simulink model "RefModel_VisualLanding"  (R2020b)
settings: Solver=ode1  StartTime=0.0  StopTime=inf  FixedStep=Ts_VisualLanding.Ts_Base  RelTol=1e-3
values from neighbouring files (symbols this model uses):
  VISLANDING_PARAM_V10 = VISLANDING_PARAM_V1000    [INIT_VisualLanding.m]    (also in SetAlgoParam_VisualLanding.m)
  VISLANDING_PARAM_V1000 = Simulink.Bus.createMATLABStruct('BUS_VISUALLANDING_PARAM')    [INIT_VisualLanding.m]    (also in SetAlgoParam_VisualLanding.m)
settings Model: PauseTimes=[308,310,12]  Creator=sl  LastModifiedBy=sl
settings DataIOCC: SaveOutput=off  SaveTime=off
settings OptimizationCC: DefaultParameterBehavior=Inlined  EnhancedBackFolding=on  PassReuseOutputArgsAs=Individual arguments  ZeroExternalMemoryAtStartup=off  ZeroInternalMemoryAtStartup=off  OptimizeBlockOrder=speed  DifferentSizesBufferReuse=on  OptimizationCustomize=off  EfficientTunableParamExpr=on
settings DebuggingCC: InheritedTsInSrcMsg=none  ParameterPrecisionLossMsg=none  ParameterTunabilityLossMsg=error  UnconnectedInputMsg=none  UnconnectedOutputMsg=none  UnconnectedLineMsg=none  SFUnusedDataAndEventsDiag=none
settings HardwareCC: ProdBitPerPointer=32  ProdBitPerSizeT=32  ProdBitPerPtrDiffT=32  ProdLargestAtomicInteger=Long  ProdLargestAtomicFloat=Double  ProdWordSize=32  ProdHWDeviceType=ARM Compatible->ARM Cortex
settings ModelReferenceCC: ModelReferenceNumInstancesAllowed=Single
settings SFSimCC: MATLABDynamicMemAlloc=off
settings RTWCC: Description=Embedded Coder  SystemTargetFile=ert.tlc  TemplateMakefile=ert_default_tmf  GenerateReport=on  IncludeHyperlinkInReport=on  LaunchReport=on  GenerateTraceInfo=on  GenerateTraceReport=on  GenerateTraceReportSl=on  GenerateTraceReportSf=on  GenerateTraceReportEml=on
settings CodeAppCC: ForceParamTrailComments=on  IgnoreCustomStorageClasses=off  MaxIdLength=48  OperatorAnnotations=on  SimulinkDataObjDesc=on  SFDataObjDesc=on  InsertBlockDesc=on
settings ERTTargetCC: TargetLangStandard=C99 (ISO)  GenerateSampleERTMain=on  CombineOutputUpdateFcns=off  LogVarNameModifier=none  SupportVariableSizeSignals=on  InlinedParameterPlacement=NonHierarchical  ERTCustomFileTemplate=example_file_process.tlc

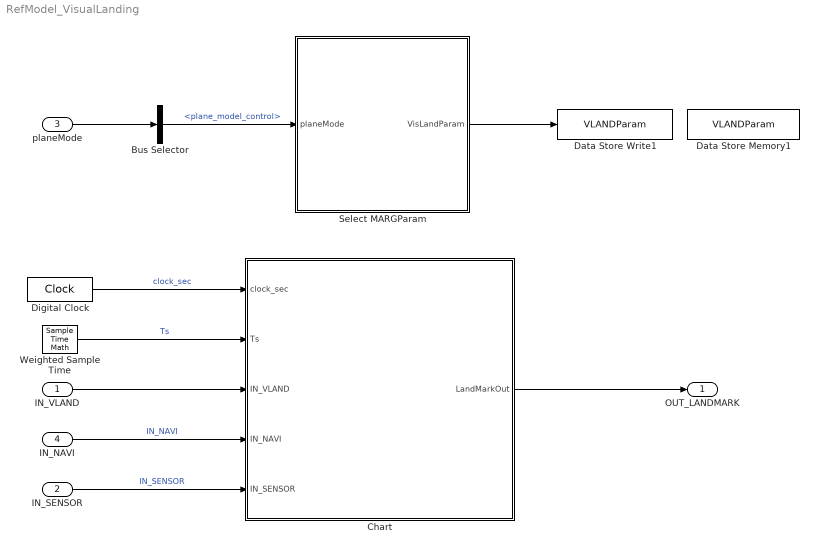
== system RefModel_VisualLanding ==
  IN_VLAND : Inport  OutDataTypeStr=Bus: BUS_VISUALLANDING_INPUT  PortDimensions=1  BusOutputAsStruct=on
  IN_SENSOR : Inport  Port=2  OutDataTypeStr=Bus: BUS_SENSOR  BusOutputAsStruct=on
  planeMode : Inport  Port=3  OutDataTypeStr=Bus: BUS_SYSTEMINFO_INPUT
  IN_NAVI : Inport  Port=4  OutDataTypeStr=Bus: BUS_NAVI_TO_FIRM  BusOutputAsStruct=on
  Bus Selector : BusSelector  OutputSignals=plane_model_control
  Chart : Stateflow chart  TreatAsAtomicUnit=on
  Data Store Memory1 : DataStoreMemory  DataStoreName=VLANDParam  ReadBeforeWriteMsg=warning  WriteAfterWriteMsg=warning  WriteAfterReadMsg=warning  ShowAdditionalParam=off  OutDataTypeStr=Bus: BUS_VISUALLANDING_PARAM  Dimensions=1
  Data Store Write1 : DataStoreWrite  DataStoreName=VLANDParam
  Digital Clock : DigitalClock  SampleTime=-1
  Select MARGParam : Subsystem
  Weighted Sample Time : SampleTimeMath  TsampMathOp=Ts Only
  OUT_LANDMARK : Outport  OutDataTypeStr=Bus: BUS_VISUALLANDING_LANDMARK
  wires:
  IN_VLAND/1 -> Chart/3(IN_VLAND)
  IN_NAVI/1 -> Chart/4(IN_NAVI)  "IN_NAVI"
  IN_SENSOR/1 -> Chart/5(IN_SENSOR)  "IN_SENSOR"
  Bus Selector/1 -> Select MARGParam/1(planeMode)  "<plane_model_control>"
  Select MARGParam/1(VisLandParam) -> Data Store Write1/1
  planeMode/1 -> Bus Selector/1
  Chart/1(LandMarkOut) -> OUT_LANDMARK/1
  Weighted Sample Time/1 -> Chart/2(Ts)  "Ts"
  Digital Clock/1 -> Chart/1(clock_sec)  "clock_sec"

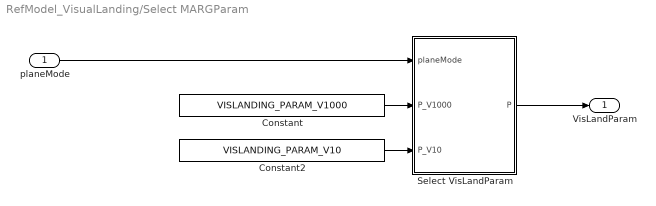
== system RefModel_VisualLanding/Select MARGParam ==
  planeMode : Inport
  Constant : Constant  Value=VISLANDING_PARAM_V1000  OutDataTypeStr=Bus: BUS_VISUALLANDING_PARAM
  Constant2 : Constant  Value=VISLANDING_PARAM_V10  OutDataTypeStr=Bus: BUS_VISUALLANDING_PARAM
  Select VisLandParam : MATLAB Function  TreatAsAtomicUnit=on
  VisLandParam : Outport
  wires:
  Constant/1 -> Select VisLandParam/2(P_V1000)
  Constant2/1 -> Select VisLandParam/3(P_V10)
  Select VisLandParam/1(P) -> VisLandParam/1
  planeMode/1 -> Select VisLandParam/1(planeMode)

== matlab function RefModel_VisualLanding/Select MARGParam/Select VisLandParam ==
  data: planeMode input Enum: ENUM_plane_mode; P output Bus: BUS_VISUALLANDING_PARAM; P_V1000 input Bus: BUS_VISUALLANDING_PARAM; P_V10 input Bus: BUS_VISUALLANDING_PARAM
function P = fcn(planeMode,P_V1000,P_V10)
switch planeMode
    case ENUM_plane_mode.V10
        P = P_V10;
    case {ENUM_plane_mode.V1000,ENUM_plane_mode.V10s}
        P = P_V1000;
    otherwise
        P = P_V1000;
end

== stateflow chart RefModel_VisualLanding/Chart ==
  state Calculate [parallel]
    en:
    initLandMarkOut();
    du:
    algebraMethod();
    if VLANDParam.enableStateEstimate
    LandMarkOut.estMode = ENUM_EstModeVisLand.StateEstimate;
    KalmanFilterMethod();
    end
    predictLLA();
    settings: executionOrder=2
  state Status [parallel]
    settings: executionOrder=1
    state updateFlag [parallel]
      en:
      du:
      updateRefreshFlag();
      settings: executionOrder=1
    state ValidFlag [parallel]
      en:
      du:
      updateVLFlag();
      settings: executionOrder=2
  data: x_out function_output; pos_landmark function_input; vel_uav function_input; pos_uav function_input; Ts_in function_input; P_out function_output; dz_out function_output; Pz_out function_output; reset function_input; reject_threshold function_input; Q function_input; R function_input; mode function_input; clock_sec input; Ts input; IN_VLAND input; IN_NAVI input; IN_SENSOR input; VLANDParam data_store_memory; LandMarkOut output Bus: BUS_VISUALLANDING_LANDMARK size=1
  function updateRefreshFlag:
    | function updateRefreshFlag
    | % 判断数据更新时刻
    | persistent lastValidIdx preIdx
    | idxAll = IN_VLAND.idxAll;
    | if isempty(lastValidIdx)
    |     lastValidIdx = idxAll;
    |     preIdx = idxAll;
    | end
    | curIdx = idxAll;
    | if preIdx ~= curIdx
    |     LandMarkOut.updateFlag = true;
    | else
    |     LandMarkOut.updateFlag = false;
    | end
    | preIdx = idxAll;
  function algebraMethod:
    | function algebraMethod
    | % c: 相机坐标系 camera
    | % l: 着陆标志坐标系 landmark
    | % b: 机体坐标系 body
    | % e: NED坐标系 
    | % cl: landing mark to camera
    | % be: ned to body
    | % cb: body to camera
    | %%
    | if IN_VLAND.nDetect ~= 0 && LandMarkOut.updateFlag% 检测到至少1个tag
    |     tcl = getTcl(IN_VLAND);
    |     [Rcl,eulerd] = getRcl(IN_VLAND); 
    |     Rcb = VLANDParam.Rcb;
    |     Rbc = Rcb';
    |     Rbe = calRbe(double(IN_NAVI.eulerd_yaw_pitch_roll)*pi/180);
    |     Rlc = Rcl';
    |     Rce = Rcb*Rbe;
    |     Rec = Rce';
    |     Rle = Rlc*Rcb*Rbe;
    |     Rel = Rle';
    | 
    |     pos_uav = double(IN_NAVI.posNED);
    |     lla_uav = IN_NAVI.lla;
    | 
    |     LandMarkOut.Rcl = Rcl;
    |     LandMarkOut.Rbl = Rbe*Rel;
    |     LandMarkOut.Rel = Rel;
    | 
    |     LandMarkOut.Pc = tcl; % 路标中心相对相机中心的位置矢量，在相机坐标系中表示
    |     
    |     LandMarkOut.Pe = Rec * LandMarkOut.Pc + pos_uav;
    |     LandMarkOut.Pb = Rbc * LandMarkOut.Pc;
    | 
    |     LandMarkOut.estMode = ENUM_EstModeVisLand.Geometry;
    |     
    |     relPosNED = Rec * LandMarkOut.Pc;
    |     dlat = 1/111e3*relPosNED(1);
    |     dlon = 1/cos(IN_NAVI.lla(1)*pi/180)/111e3*relPosNED(2);
    |     dh = -relPosNED(3);
    |     LandMarkOut.LLA = lla_uav + [dlat;dlon;dh];
    | end
    | end
    | % LandMarkOut.Ve = [0;0;0];
    | %%
    | % 计算Rbe
    | function out = calRbe(euler_yaw_pitch_roll)
    | yaw_be = euler_yaw_pitch_roll(1);
    | pitch_be = euler_yaw_pitch_roll(2);
    | roll_be = euler_yaw_pitch_roll(3);
    | out = Rzyx(yaw_be,pitch_be,roll_be);
    | end
    | % 计算平均tcl
    | function tcl = getTcl(IN_VLAND)
    | if IN_VLAND.Tagl.isDetect
    |     tcl = IN_VLAND.Tagl.tcl;
    | elseif IN_VLAND.Tagm.isDetect
    |     tcl = IN_VLAND.Tagm.tcl; 
    | else
    |     tcl = IN_VLAND.Tags.tcl;
    | end
    | end
    | % 计算平均Rcl
    | function [Rcl,eulerd] = getRcl(IN_VLAND)
    | if IN_VLAND.Tagl.isDetect
    |     Rcl = IN_VLAND.Tagl.Rcl;
    |     eulerd = IN_VLAND.Tagl.eulerdcl;
    | elseif IN_VLAND.Tagm.isDetect
    |     Rcl = IN_VLAND.Tagm.Rcl; 
    |     eulerd = IN_VLAND.Tagl.eulerdcl;
    | else
    |     Rcl = IN_VLAND.Tags.Rcl;
    |     eulerd = IN_VLAND.Tagl.eulerdcl;
    | end
    | % Rcl = double(Rcl);
    | % eulerd = double(eulerd);
    | end
  function [x_out,P_out,dz_out,Pz_out] = landmarkKF(pos_landmark, vel_uav, pos_uav, Ts_in,reset,reject_threshold,Q,R,mode):
    | function [x_out,P_out,dz_out,Pz_out] = landmarkKF(pos_landmark, vel_uav, pos_uav, Ts_in,reset,reject_threshold,Q,R,mode)
    | persistent x P dz Pz
    | pos_landmark0 = reshape(pos_landmark,[3,1]);
    | if isempty(x) || reset
    |     vel_landmark0 = [0;0;0];
    |     state0 = [pos_landmark0;vel_landmark0];
    |     x = state0;
    |     P = diag([3^2*ones(3,1);10^2*ones(3,1);]);
    |     
    |     dz = zeros(3,1);
    |     Pz = zeros(3,3);
    | end
    | 
    | switch mode
    |     case 'predict'
    |         % 预测
    |         u = [0;0;0];
    |         [x,P] = predict(x,u,Ts_in,P,Q);
    |     otherwise % 'fuse'
    |         % 矫正
    |         z = pos_landmark;
    |         [x,P,dz,Pz] = fusePos(x,z,P,R,reject_threshold);
    | end
    | x_out = x;
    | P_out = P;
    | dz_out = dz;
    | Pz_out = Pz;
    | %%
    | % 测量
    | function [z,H] = measure(x)
    | pos_lm = x(1:3);
    | z = pos_lm;
    | H = [1 0 0  0 0 0;
    |      0 1 0  0 0 0;
    |      0 0 1  0 0 0];
    | % 预测
    | function [x,P] = predict(x,u,Ts,P,Q)
    | pos_lm = x(1:3);
    | vel_lm = x(4:6);
    | pos_lm = pos_lm + vel_lm*Ts;
    | vel_lm = vel_lm + u;
    | x = [pos_lm;vel_lm];
    | A = [zeros(3,3)   eye(3,3);
    |      zeros(3,3) zeros(3,3);];
    | PHI = eye(6) + A*Ts;
    | P = PHI*P*PHI' + Q*Ts;
    | % 校正
    | function [x,P,dz,Pz] = fusePos(x,z,P,R,reject_threshold)
    | [z_prop,H] = measure(x);
    | dz = z - z_prop;
    | Pz = H*P*H'+R;
    | % if abs(dz) < reject_threshold
    |     % 残差小于阈值
    |     K = P*H'/(H*P*H'+R);
    |     P = (eye(size(K,1))-K*H)*P;
    |     P = (P+P')/2;
    |     x = x + K*dz;
    | % else
    | %     % 残差超限拒绝测量值
    | %     x = x;
    | %     P = P;
    | % end
  function updateVLFlag:
    | function updateVLFlag
    | % 更新视觉计算
    | persistent lastValidIdx preIdx sumInvalidIdx
    | idxAll = IN_VLAND.idxAll;
    | validFlag = IN_VLAND.validFlag;
    | frameRate = IN_VLAND.frameRate;
    | if isempty(lastValidIdx)
    |     lastValidIdx = idxAll;
    |     preIdx = idxAll;
    |     sumInvalidIdx = 0;
    | end
    | curIdx = idxAll;
    | if preIdx ~= curIdx
    |     updateFlag = true;
    | else
    |     updateFlag = false;
    | end
    | preIdx = idxAll;
    | if updateFlag % 当更新帧时进行一次检测有效性判定
    |     if ~validFlag
    |         sumInvalidIdx = sumInvalidIdx + 1;
    |     else
    |         sumInvalidIdx = 0;
    |     end
    | end
    | timeTh = 3*frameRate;
    | if sumInvalidIdx >= timeTh % 当连续出现N次检测不到tag时，认为跟踪失败
    |     LandMarkOut.validFlag = false;
    | else
    |     LandMarkOut.validFlag = true;
    | end
  function predictLLA:
    | function predictLLA
    | % 根据速度进行纬度、经度外推，高度不外推
    | if LandMarkOut.validFlag
    |     dposn_m = LandMarkOut.Ve(1)*Ts;
    |     dpose_m = LandMarkOut.Ve(2)*Ts;
    |     dlat = 1/111e3*dposn_m;
    |     dlon = 1/cos(IN_NAVI.lla(1)*pi/180)/111e3*dpose_m;
    |     dh = 0;
    |     LandMarkOut.LLA = LandMarkOut.LLA + [dlat;dlon;dh];
    | end
  function KalmanFilterMethod:
    | function KalmanFilterMethod
    | % persistent dz x P Pz
    | % if isempty(dz) ||...
    | %         ~LandMarkOut.validFlag % Tag跟踪丢失
    | %     dz = 0;
    | %     x = 0;
    | %     P = diag([]);
    | %     Pz = 0;
    | % end
    | persistent preValidFlag
    | if isempty(preValidFlag)
    |     preValidFlag = false;
    | end
    | if ~preValidFlag && LandMarkOut.validFlag
    |     resetKF = true;
    | else
    |     resetKF = false;
    | end
    | preValidFlag = LandMarkOut.validFlag;
    | %%
    | if LandMarkOut.validFlag
    |     pos_uav = double(IN_NAVI.posNED);
    |     vel_uav = double(IN_NAVI.velNED);
    |     pos_landmark = LandMarkOut.Pe;
    | 
    |     R = diag([1*ones(3,1)].^2); % 高度测量偏差
    |     sigma_pos_ml = 0.1*ones(3,1);
    |     sigma_vel_ml = 3*ones(3,1);
    |     Q = diag([sigma_pos_ml;sigma_vel_ml;].^2);
    |     reject_threshold = 0;
    |     % [x,P,dz,Pz] = landmarkKF(Vd,heightRadar1,Ts,resetKF,reject_threshold,Q,R,'predict');
    |     [x,P,dz,Pz] = landmarkKF(pos_landmark, vel_uav, pos_uav, Ts,resetKF,reject_threshold,Q,R,'predict');
    |     if LandMarkOut.updateFlag
    |         [x,P,dz,Pz] = landmarkKF(pos_landmark, vel_uav, pos_uav, Ts,resetKF,reject_threshold,Q,R,'fuse');
    |     end
    |     LandMarkOut.Pe = x(1:3);
    |     LandMarkOut.Ve = x(4:6);
    |     LandMarkOut.posCov = diag(P(1:3,1:3));
    |     LandMarkOut.velCov = diag(P(4:6,4:6));
    | else
    |     LandMarkOut.Ve = [0;0;0];
    | end
  function initLandMarkOut:
    | function initLandMarkOut
    | LandMarkOut.Rcl = zeros(3);
    | LandMarkOut.Rbl = zeros(3);
    | LandMarkOut.Rel = zeros(3);
    | 
    | LandMarkOut.LLA = zeros(3,1);
    | LandMarkOut.Pe = zeros(3,1);
    | LandMarkOut.Ve = zeros(3,1);
    | LandMarkOut.Pc = zeros(3,1); % 路标中心相对相机中心的位置矢量，在相机坐标系中表示
    | LandMarkOut.Pb = zeros(3,1);
    | LandMarkOut.posCov = zeros(3,1);
    | LandMarkOut.velCov = zeros(3,1);
    | LandMarkOut.estMode = ENUM_EstModeVisLand.Geometry;
    | LandMarkOut.validFlag = false;
    | LandMarkOut.updateFlag = false;
